simulink model "City_Environment_CS2020"  (Simulink 8.8)
settings: Solver=ode45  StartTime=0  StopTime=25  RelTol=1e-3  EnableMultiTasking=on
libraries: Solver_SF x4
settings Model: Creator=dhall  LastModifiedBy=mkhan  ExtModeTrigMode=oneshot  ExtModeArmWhenConnect=off
settings DataIOCC: LimitDataPoints=off  SignalLoggingName=sigsOut
settings OptimizationCC: BooleanDataType=off  LocalBlockOutputs=off  InitFltsAndDblsToZero=on
settings DebuggingCC: SaveWithParameterizedLinksMsg=none  SignalResolutionControl=TryResolveAllWithWarning  MultiTaskDSMMsg=warning  MultiTaskCondExecSysMsg=none  SFExecutionAtInitializationDiag=warning
settings HardwareCC: TargetBitPerPointer=64  TargetBitPerSizeT=64  TargetBitPerPtrDiffT=64  TargetLongLongMode=on  TargetIntDivRoundTo=Zero  TargetEndianess=LittleEndian  TargetWordSize=64  TargetHWDeviceType=MATLAB Host  ProdEqTarget=off
settings GRTTargetCC: TargetFcnLib=ansi_tfl_tmw.mat  CompOptLevelCompliant=off
settings ConfigComp: CovSFcnEnable=off

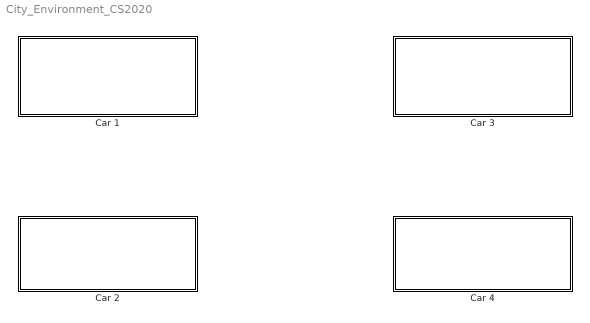
== system City_Environment_CS2020 ==
  Car 1 : Subsystem
  Car 2 : Subsystem
  Car 3 : Subsystem
  Car 4 : Subsystem

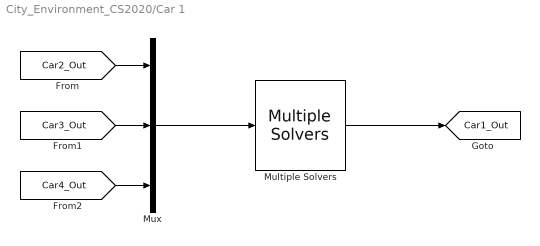
== system City_Environment_CS2020/Car 1 ==
  Multiple Solvers : Solver_SF/Multiple Solvers  Priority=1  iVehicle=1  SIMFILE=D:\CarSim2020.0\CarSim_Data\simfile1.sim  Run_RTs=off  vs_state_ind=Run  StopMode_ind=Vehicle Model  vs_scx=on
  Mux : Mux  Inputs=3
  tag scope: Car1_Out=global
  wires:
  Multiple Solvers/1 -> [Car1_Out]
  Mux/1 -> Multiple Solvers/1
  [Car2_Out] -> Mux/1
  [Car3_Out] -> Mux/2
  [Car4_Out] -> Mux/3

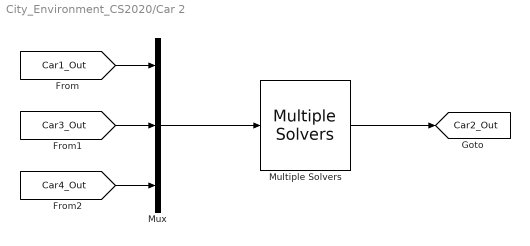
== system City_Environment_CS2020/Car 2 ==
  Multiple Solvers : Solver_SF/Multiple Solvers  Priority=1  iVehicle=2  SIMFILE=D:\CarSim2020.0\CarSim_Data\simfile2.sim  Run_RTs=off  vs_state_ind=Run  StopMode_ind=Vehicle Model  vs_scx=on
  Mux : Mux  Inputs=3
  tag scope: Car2_Out=global
  wires:
  Mux/1 -> Multiple Solvers/1
  Multiple Solvers/1 -> [Car2_Out]
  [Car1_Out] -> Mux/1
  [Car3_Out] -> Mux/2
  [Car4_Out] -> Mux/3

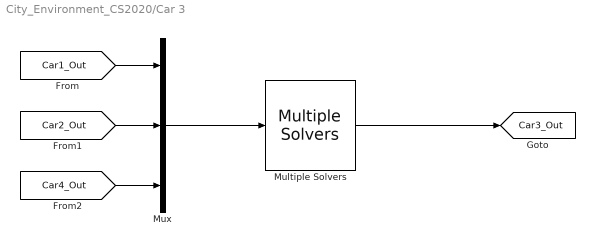
== system City_Environment_CS2020/Car 3 ==
  Multiple Solvers : Solver_SF/Multiple Solvers  Priority=1  iVehicle=3  SIMFILE=D:\CarSim2020.0\CarSim_Data\simfile3.sim  Run_RTs=off  vs_state_ind=Run  StopMode_ind=Vehicle Model  vs_scx=on
  Mux : Mux  Inputs=3
  tag scope: Car3_Out=global
  wires:
  Multiple Solvers/1 -> [Car3_Out]
  Mux/1 -> Multiple Solvers/1
  [Car1_Out] -> Mux/1
  [Car2_Out] -> Mux/2
  [Car4_Out] -> Mux/3

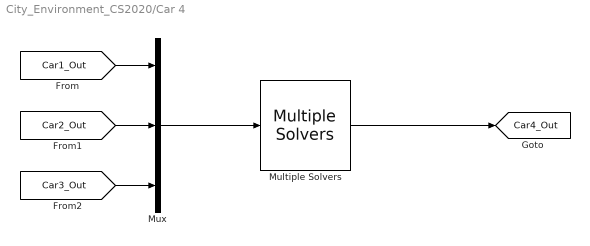
== system City_Environment_CS2020/Car 4 ==
  Multiple Solvers : Solver_SF/Multiple Solvers  Priority=1  iVehicle=4  SIMFILE=D:\CarSim2020.0\CarSim_Data\simfile4.sim  Run_RTs=off  vs_state_ind=Run  StopMode_ind=Vehicle Model  vs_scx=on
  Mux : Mux  Inputs=3
  tag scope: Car4_Out=global
  wires:
  Multiple Solvers/1 -> [Car4_Out]
  Mux/1 -> Multiple Solvers/1
  [Car1_Out] -> Mux/1
  [Car2_Out] -> Mux/2
  [Car3_Out] -> Mux/3
